simulink model "HFV_model_updated"  (R2019b)
settings: Solver=VariableStepAuto  StartTime=0.0  StopTime=10  FixedStep=0.  RelTol=1e-3
libraries: simulink x1
settings Model: Creator=114-AO  LastModifiedBy=114-AO
settings DebuggingCC: UnderSpecifiedDimensionMsg=warning

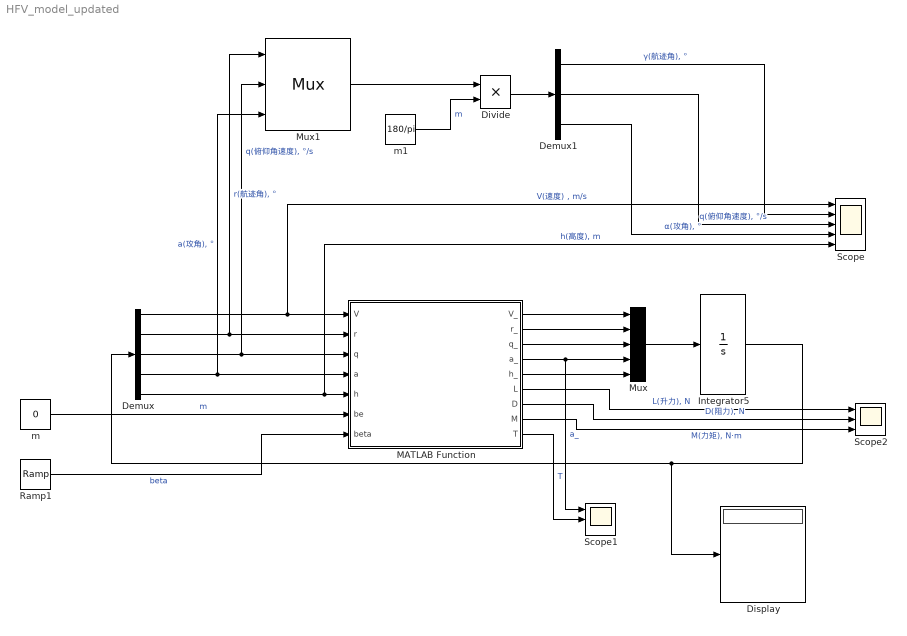
== system HFV_model_updated ==
  Demux : Demux  Outputs=5
  Demux1 : Demux  Outputs=3
  Display : Display
  Divide : Product  Inputs=**
  Integrator5 : Integrator  InitialCondition=[4590.3, 0*pi/180, 0*pi/180, 2.745*pi/180, 33528]
  MATLAB Function : MATLAB Function  TreatAsAtomicUnit=on
  Mux : Mux  Inputs=5
      settings: DisplayOption=signals
  Mux1 : Mux  Inputs=3
      settings: DisplayOption=signals
  Ramp1 : simulink/Sources/Ramp  slope=0  start=0  InitialOutput=0
  Scope : Scope  NumInputPorts=5
  Scope1 : Scope  NumInputPorts=3
  Scope2 : Scope  NumInputPorts=3
  m : Constant  Value=0
  m1 : Constant  Value=180/pi
  wires:
  Mux/1 -> Integrator5/1
  MATLAB Function/1(V_) -> Mux/1
  MATLAB Function/4(a_) -> Scope1/1, Mux/4  "a_"
  MATLAB Function/5(h_) -> Mux/5
  MATLAB Function/2(r_) -> Mux/2
  MATLAB Function/3(q_) -> Mux/3
  Integrator5/1 -> Display/1, Demux/1
  Demux/1 -> Scope/1, MATLAB Function/1(V)  "V(速度)，m/s"
  Demux/2 -> MATLAB Function/2(r), Mux1/1  "r(航迹角), °"
  Demux/5 -> MATLAB Function/5(h), Scope/5  "h(高度), m"
  Demux/4 -> MATLAB Function/4(a), Mux1/3  "a(攻角), °"
  m/1 -> MATLAB Function/6(be)  "m"
  Ramp1/1 -> MATLAB Function/7(beta)  "beta"
  MATLAB Function/6(L) -> Scope2/1  "L(升力), N"
  MATLAB Function/7(D) -> Scope2/2  "D(阻力), N"
  MATLAB Function/8(M) -> Scope2/3  "M(力矩), N·m"
  Demux/3 -> MATLAB Function/3(q), Mux1/2  "q(俯仰角速度), °/s"
  MATLAB Function/9(T) -> Scope1/2  "T"
  Mux1/1 -> Divide/1
  Divide/1 -> Demux1/1
  Demux1/1 -> Scope/2  "γ(航迹角), °"
  Demux1/2 -> Scope/3  "q(俯仰角速度), °/s"
  Demux1/3 -> Scope/4  "α(攻角), °"
  m1/1 -> Divide/2  "m"

== matlab function HFV_model_updated/MATLAB Function ==
  data: V input; r input; q input; V_ output; r_ output; q_ output; a input; h input; be input; beta input; a_ output; h_ output; L output; D output; M output; T output
function [V_, r_, q_, a_, h_, L, D, M, T] = HFVParams(V, r, q, a, h, be, beta)

%% 参数
m = 136820;
Iyy = 9490740;
S = 334.73;
c_ = 24.38;
rho0 = 1.2266;
rho = rho0*exp(-h/7315.2);
g0 = 9.80665;
r0 = 6356766;
g = g0*(r0/(r0+h))^2;
ce = 0.0292;
q__ = 0.5*rho*V^2;


%% 气动力
L = q__*S*0.6203*a;
D = q__*S*(0.6450*a^2 + 0.0043378*a + 0.003772);
CMa = -0.035*a^2 + 0.036617*a + 5.3261*10^(-6);
CMq = 0.5*c_*q*(-6.796*a^2 + 0.3015*a - 0.2289) / V;
CMbe = ce*(be - a);
M = q__*S*c_*(CMa + CMq + CMbe);% M = 1;

%% 推力
if(beta<1) 
    CT = 0.02579*beta;
else
    CT = 0.0224 +0.00336*beta;
end
T = q__* S * CT;

%% 运动方程
V_ = (T*cos(a) - D)/m - g*sin(r);
r_ = (L + T*sin(a))/(m*V) - g*cos(r)/V;
q_ = M/Iyy;

a_ = q - r_;
h_ = V*sin(r);

% V_ = (T*cos(a) - D)/m - g*sin(r);
% r_ = (L + T*sin(a))/(m*V) - g*cos(r)/V;
% q_ = M/Iyy;
% a_ = q - r_;
% h_ = V*sin(r);


end
